simulink model "Einfache_Zustandsrueckfuehrung_nichtlinear"  (R2022a)
settings: Solver=FixedStepAuto  StartTime=0.0  StopTime=5  FixedStep=1/1e4  RelTol=1e-3
undefined symbols (not defined in the file): c, k, Phi, Phi_Punkt, start_deg, Theta, Theta_Punkt, V_m, x_c
settings Model: Creator=basti  LastModifiedBy=milan
settings DataIOCC: ReturnWorkspaceOutputsName=SDOSimTest_Log
settings DebuggingCC: UnconnectedInputMsg=warning  UnconnectedOutputMsg=warning  UnconnectedLineMsg=warning
settings RTWCC: DLArmComputeVersion=19.05

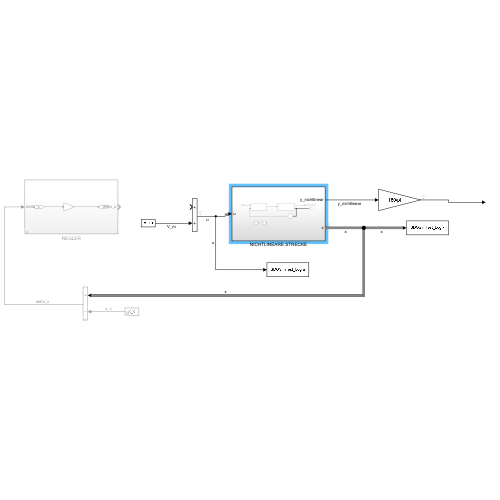
[thumbnail: Simulink's stored preview of the top-level diagram]
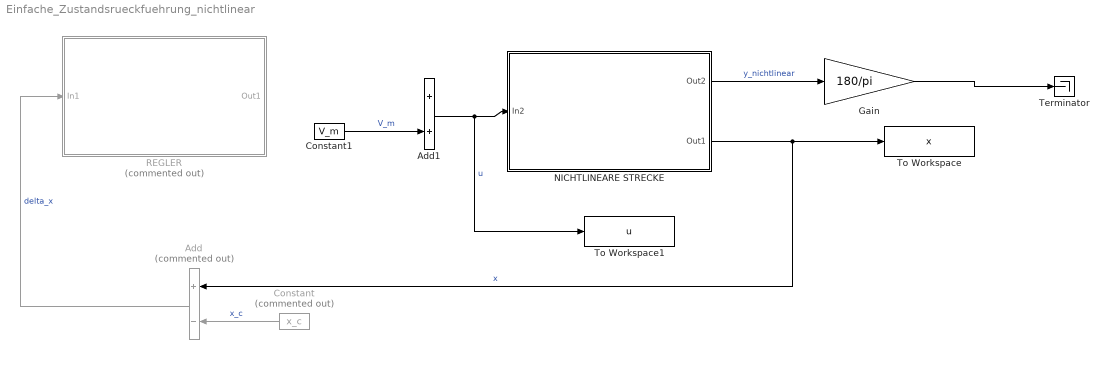
== system Einfache_Zustandsrueckfuehrung_nichtlinear ==
  Add : Sum  Commented=on  Inputs=+-
  Add1 : Sum
  Constant : Constant  Commented=on  Value=x_c
  Constant1 : Constant  Value=V_m  VectorParams1D=off
  Gain : Gain  Gain=180/pi
  NICHTLINEARE STRECKE : Subsystem
  REGLER : Subsystem  Commented=on
  Terminator : Terminator
  To Workspace : ToWorkspace  VariableName=x  SaveFormat=Timeseries  SampleTime=-1
  To Workspace1 : ToWorkspace  VariableName=u  SaveFormat=Timeseries  SampleTime=-1
  wires:
  NICHTLINEARE STRECKE/1(Out2) -> Gain/1  "y_nichtlinear"
  Constant/1 -> Add/2  "x_c"
  NICHTLINEARE STRECKE/2(Out1) -> Add/1, To Workspace/1  "x"
  Add/1 -> REGLER/1(In1)  "delta_x"
  Add1/1 -> To Workspace1/1, NICHTLINEARE STRECKE/1(In2)  "u"
  Constant1/1 -> Add1/2  "V_m"
  Gain/1 -> Terminator/1

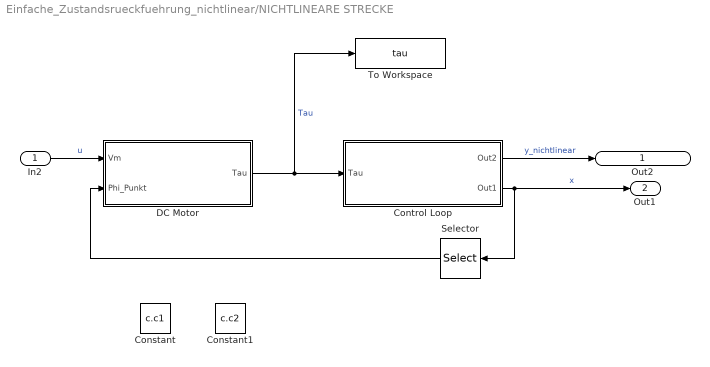
== system Einfache_Zustandsrueckfuehrung_nichtlinear/NICHTLINEARE STRECKE ==
  In2 : Inport
  Constant : Constant  Value=c.c1
  Constant1 : Constant  Value=c.c2
  Control Loop : Subsystem
  DC Motor : Subsystem
  Selector : Selector  InputPortWidth=4  IndexOptions=Index vector (dialog)  Indices=4  OutputSizes=1
  To Workspace : ToWorkspace  VariableName=tau  SaveFormat=Timeseries  SampleTime=-1
  Out2 : Outport
  Out1 : Outport  Port=2
  wires:
  In2/1 -> DC Motor/1(Vm)  "u"
  DC Motor/1(Tau) -> To Workspace/1, Control Loop/1(Tau)  "Tau"
  Control Loop/2(Out1) -> Out1/1, Selector/1  "x"
  Selector/1 -> DC Motor/2(Phi_Punkt)
  Control Loop/1(Out2) -> Out2/1  "y_nichtlinear"

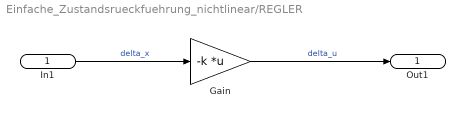
== system Einfache_Zustandsrueckfuehrung_nichtlinear/REGLER ==
  In1 : Inport
  Gain : Gain  Gain=-k  Multiplication=Matrix(K*u) (u vector)
  Out1 : Outport
  wires:
  Gain/1 -> Out1/1  "delta_u"
  In1/1 -> Gain/1  "delta_x"

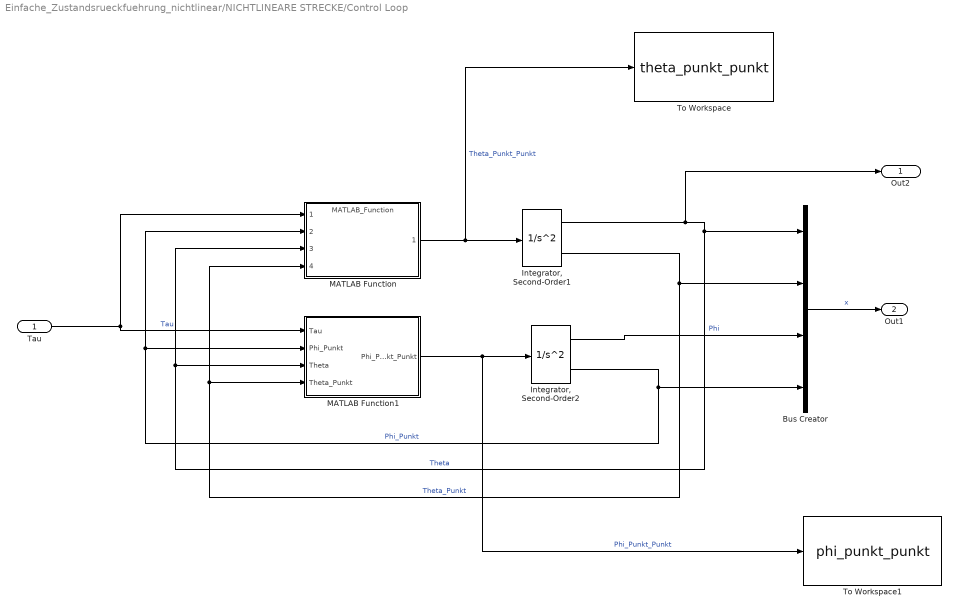
== system Einfache_Zustandsrueckfuehrung_nichtlinear/NICHTLINEARE STRECKE/Control Loop ==
  Tau : Inport
  Bus Creator : BusCreator  Inputs=Theta,Theta_Punkt,Phi,Phi_Punkt
  "Integrator, Second-Order1" : SecondOrderIntegrator  ICX=x_c(1)+(start_deg*pi/180)  ICDXDT=x_c(2)
  "Integrator, Second-Order2" : SecondOrderIntegrator  ICX=x_c(3)  ICDXDT=x_c(4)
  MATLAB Function : ModelReference  ModelNameDialog=MATLAB_Function  SimulationMode=Normal  ModelReferenceVersion=2.4
  MATLAB Function1 : MATLAB Function  TreatAsAtomicUnit=on
  To Workspace : ToWorkspace  VariableName=theta_punkt_punkt  SaveFormat=Timeseries  SampleTime=-1
  To Workspace1 : ToWorkspace  VariableName=phi_punkt_punkt  SaveFormat=Timeseries  SampleTime=-1
  Out2 : Outport
  Out1 : Outport  Port=2
  wires:
  MATLAB Function/1 -> To Workspace/1, "Integrator, Second-Order1"/1  "Theta_Punkt_Punkt"
  MATLAB Function1/1(Phi_Punkt_Punkt) -> To Workspace1/1, "Integrator, Second-Order2"/1  "Phi_Punkt_Punkt"
  "Integrator, Second-Order2"/2 -> MATLAB Function/2, MATLAB Function1/2(Phi_Punkt), Bus Creator/4  "Phi_Punkt"
  "Integrator, Second-Order1"/1 -> Out2/1, MATLAB Function/3, MATLAB Function1/3(Theta), Bus Creator/1  "Theta"
  "Integrator, Second-Order1"/2 -> MATLAB Function/4, MATLAB Function1/4(Theta_Punkt), Bus Creator/2  "Theta_Punkt"
  Tau/1 -> MATLAB Function/1, MATLAB Function1/1(Tau)  "Tau"
  "Integrator, Second-Order2"/1 -> Bus Creator/3  "Phi"
  Bus Creator/1 -> Out1/1  "x"

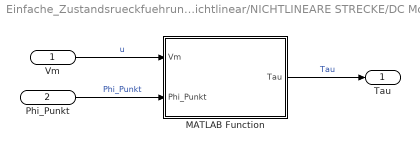
== system Einfache_Zustandsrueckfuehrung_nichtlinear/NICHTLINEARE STRECKE/DC Motor ==
  Vm : Inport
  Phi_Punkt : Inport  Port=2
  MATLAB Function : MATLAB Function  TreatAsAtomicUnit=on
  Tau : Outport
  wires:
  Vm/1 -> MATLAB Function/1(Vm)  "u"
  Phi_Punkt/1 -> MATLAB Function/2(Phi_Punkt)  "Phi_Punkt"
  MATLAB Function/1(Tau) -> Tau/1  "Tau"

== matlab function Einfache_Zustandsrueckfuehrung_nichtlinear/NICHTLINEARE STRECKE/Control Loop/MATLAB Function1 ==
  data: Tau input; Phi_Punkt_Punkt output; Phi_Punkt input; Theta input; Theta_Punkt input; c parameter
function Phi_Punkt_Punkt = fcn(Tau, Phi_Punkt, Theta, Theta_Punkt,c)
    % Konstanten aufrufen
     %c = Konstanten();
    
    % Berechnung
        Phi_Punkt_Punkt = (((c.m1*c.l1+c.m2*c.l2)*c.g*sin(Theta)-c.c1*Theta_Punkt-(c.m1*c.l1^2+c.m2*c.l2^2+c.J1+c.J2)*(Tau-c.c2*Phi_Punkt)/c.J2)/c.J2)/(1-(c.m1*c.l1^2+c.m2*c.l2^2+c.J1+c.J2)/c.J2);

== matlab function Einfache_Zustandsrueckfuehrung_nichtlinear/NICHTLINEARE STRECKE/DC Motor/MATLAB Function ==
  data: Vm input; Tau output; Phi_Punkt input
function Tau = fcn(Vm, Phi_Punkt)
    % Konstanten
    c = Konstanten();
    
    % Berechnung
    Tau = c.Kt*(Vm-c.Kb*Phi_Punkt)/c.Ra;
